simulink model "Correlation"  (R2012b)
settings: Solver=ode45  StartTime=0.0  StopTime=1280e-9  RelTol=1e-3
undefined symbols (not defined in the file or in its folder): Radix
libraries: dspxfrm3 x6
settings Model: Creator=Ahmad  LastModifiedBy=Ahmad

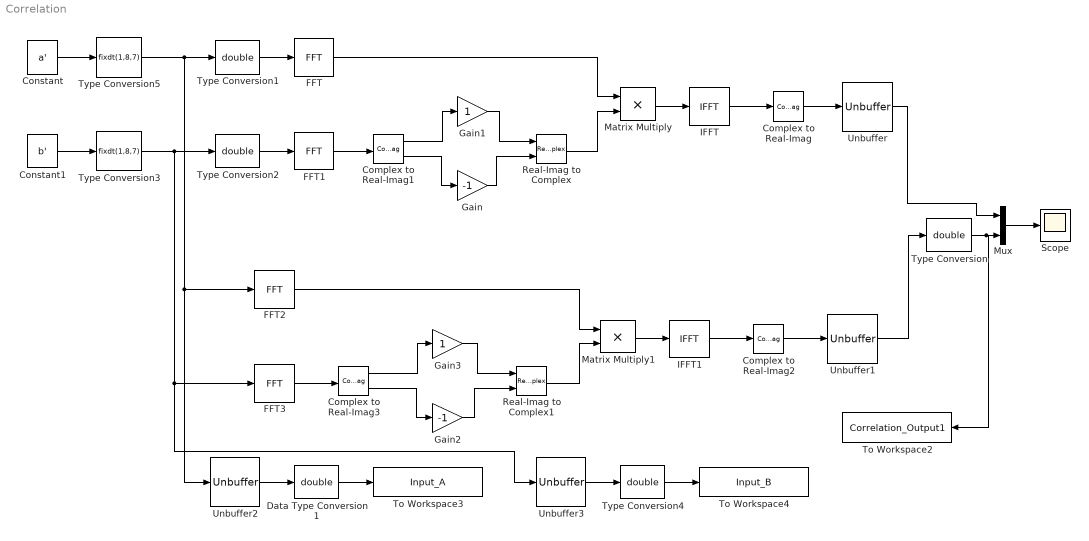
== system Correlation ==
  Complex to Real-Imag : ComplexToRealImag  Output=Real
  Complex to Real-Imag1 : ComplexToRealImag
  Complex to Real-Imag2 : ComplexToRealImag  Output=Real
  Complex to Real-Imag3 : ComplexToRealImag
  Constant : Constant  Value=a'  VectorParams1D=off  OutDataTypeStr=double  SampleTime=1/100e6  FramePeriod=128/100e6
      settings: SamplingMode=Frame based
  Constant1 : Constant  Value=b'  VectorParams1D=off  OutDataTypeStr=double  SampleTime=1/100e6  FramePeriod=128/100e6
      settings: SamplingMode=Frame based
  Data Type Conversion1 : DataTypeConversion  OutDataTypeStr=double
  FFT : dspxfrm3/FFT  CompMethod=Table lookup  TableOpt=NEW  TableOptActive=Speed  BitRevOrder=off  InheritFFTLength=off  FFTLength=128  RowConvenienceOn=on  FFTImplementation=Radix-2  SkipNorm=off  firstCoeffDataTypeStr=Inherit: Same word length as input  firstCoeffLastDataTypeStr=Inherit: Same word length as input  outputMin=[]  outputMax=[]  roundingMode=Floor  overflowMode=off
  FFT1 : dspxfrm3/FFT  CompMethod=Table lookup  TableOpt=NEW  TableOptActive=Speed  BitRevOrder=off  InheritFFTLength=off  FFTLength=128  RowConvenienceOn=on  FFTImplementation=Radix-2  SkipNorm=off  firstCoeffDataTypeStr=Inherit: Same word length as input  firstCoeffLastDataTypeStr=Inherit: Same word length as input  outputMin=[]  outputMax=[]  roundingMode=Floor  overflowMode=off
  FFT2 : dspxfrm3/FFT  CompMethod=Table lookup  TableOpt=NEW  TableOptActive=Speed  BitRevOrder=off  InheritFFTLength=off  FFTLength=128  RowConvenienceOn=on  FFTImplementation=Radix-2  SkipNorm=off  firstCoeffMode=Specify word length  firstCoeffWordLength=8  firstCoeffFracLength=15  firstCoeffDataTypeStr=fixdt(1,8)  firstCoeffLastDataTypeStr=fixdt(1,8)  outputMode=Binary point scaling  outputWordLength=16  outputFracLength=7  outputDataTypeStr=fixdt(1,16,7)  outputLastDataTypeStr=fixdt(1,16,7)  outputMin=[]  outputMax=[]  accumMode=Binary point scaling  accumWordLength=16  accumFracLength=7  accumDataTypeStr=fixdt(1,16,7)  accumLastDataTypeStr=fixdt(1,16,7)  prodOutputMode=Binary point scaling  prodOutputWordLength=11  prodOutputFracLength=7  prodOutputDataTypeStr=fixdt(1,11,7)  prodOutputLastDataTypeStr=fixdt(1,11,7)  roundingMode=Floor  overflowMode=off
  FFT3 : dspxfrm3/FFT  CompMethod=Table lookup  TableOpt=NEW  TableOptActive=Speed  BitRevOrder=off  InheritFFTLength=off  FFTLength=128  RowConvenienceOn=on  FFTImplementation=Radix-2  SkipNorm=off  firstCoeffMode=Specify word length  firstCoeffWordLength=8  firstCoeffFracLength=15  firstCoeffDataTypeStr=fixdt(1,8)  firstCoeffLastDataTypeStr=fixdt(1,8)  outputMode=Binary point scaling  outputWordLength=16  outputFracLength=7  outputDataTypeStr=fixdt(1,16,7)  outputLastDataTypeStr=fixdt(1,16,7)  outputMin=[]  outputMax=[]  accumMode=Binary point scaling  accumWordLength=16  accumFracLength=7  accumDataTypeStr=fixdt(1,16,7)  accumLastDataTypeStr=fixdt(1,16,7)  prodOutputMode=Binary point scaling  prodOutputWordLength=11  prodOutputFracLength=7  prodOutputDataTypeStr=fixdt(1,11,7)  prodOutputLastDataTypeStr=fixdt(1,11,7)  roundingMode=Floor  overflowMode=off
  Gain : Gain  Gain=-1
  Gain1 : Gain
  Gain2 : Gain  Gain=-1  OutDataTypeStr=fixdt(1,16,7)
  Gain3 : Gain  OutDataTypeStr=fixdt(1,16,7)
  IFFT : dspxfrm3/IFFT  CompMethod=Table lookup  TableOpt=NEW  TableOptActive=Speed  BitRevOrder=off  cs_in=off  SkipNorm=off  InheritFFTLength=off  FFTLength=128  mode=Complex  outSamplingMode=Frame based  RowConvenienceOn=on  FFTImplementation=Radix-2  firstCoeffDataTypeStr=Inherit: Same word length as input  firstCoeffLastDataTypeStr=Inherit: Same word length as input  outputMin=[]  outputMax=[]  roundingMode=Floor  overflowMode=off
  IFFT1 : dspxfrm3/IFFT  CompMethod=Table lookup  TableOpt=NEW  TableOptActive=Speed  BitRevOrder=off  cs_in=off  SkipNorm=off  InheritFFTLength=off  FFTLength=128  mode=Complex  outSamplingMode=Frame based  RowConvenienceOn=on  FFTImplementation=Radix-2  firstCoeffMode=Specify word length  firstCoeffWordLength=16  firstCoeffFracLength=15  firstCoeffDataTypeStr=fixdt(1,16)  firstCoeffLastDataTypeStr=fixdt(1,16)  outputMode=Binary point scaling  outputWordLength=33  outputFracLength=7  outputDataTypeStr=fixdt(1,33,7)  outputLastDataTypeStr=fixdt(1,33,7)  outputMin=[]  outputMax=[]  accumMode=Binary point scaling  accumWordLength=33  accumFracLength=7  accumDataTypeStr=fixdt(1,33,7)  accumLastDataTypeStr=fixdt(1,33,7)  prodOutputMode=Binary point scaling  prodOutputWordLength=25  prodOutputFracLength=7  prodOutputDataTypeStr=fixdt(1,25,7)  prodOutputLastDataTypeStr=fixdt(1,25,7)  roundingMode=Floor  overflowMode=off
  Matrix Multiply : Product
  Matrix Multiply1 : Product  OutDataTypeStr=fixdt(1,25,7)
  Mux : Mux  Inputs=2
  Real-Imag to Complex : RealImagToComplex
  Real-Imag to Complex1 : RealImagToComplex
  Scope : Scope
      settings: YMin=0.1  YMax=0.85
  To Workspace2 : ToWorkspace  VariableName=Correlation_Output1  SampleTime=-1  SaveFormat=Timeseries
  To Workspace3 : ToWorkspace  VariableName=Input_A  SampleTime=-1  SaveFormat=Timeseries
  To Workspace4 : ToWorkspace  VariableName=Input_B  SampleTime=-1  SaveFormat=Timeseries
  Type Conversion{,1..2,4} (4 alike) : DataTypeConversion  OutDataTypeStr=double
  Type Conversion3 : DataTypeConversion  OutDataTypeStr=fixdt(1,8,7)
  Type Conversion5 : DataTypeConversion  OutDataTypeStr=fixdt(1,8,7)
  Unbuffer{,1..3} (4 alike) : Unbuffer
  wires:
  Complex to Real-Imag/1 -> Unbuffer/1
  IFFT/1 -> Complex to Real-Imag/1
  FFT1/1 -> Complex to Real-Imag1/1
  Complex to Real-Imag1/1 -> Gain1/1
  Complex to Real-Imag1/2 -> Gain/1
  Gain1/1 -> Real-Imag to Complex/1
  Gain/1 -> Real-Imag to Complex/2
  FFT/1 -> Matrix Multiply/1
  Real-Imag to Complex/1 -> Matrix Multiply/2
  Matrix Multiply/1 -> IFFT/1
  Constant/1 -> Type Conversion5/1
  Constant1/1 -> Type Conversion3/1
  Unbuffer/1 -> Mux/1
  Complex to Real-Imag2/1 -> Unbuffer1/1
  IFFT1/1 -> Complex to Real-Imag2/1
  FFT3/1 -> Complex to Real-Imag3/1
  Complex to Real-Imag3/1 -> Gain3/1
  Complex to Real-Imag3/2 -> Gain2/1
  Gain3/1 -> Real-Imag to Complex1/1
  Gain2/1 -> Real-Imag to Complex1/2
  FFT2/1 -> Matrix Multiply1/1
  Matrix Multiply1/1 -> IFFT1/1
  Unbuffer1/1 -> Type Conversion/1
  Mux/1 -> Scope/1
  Type Conversion/1 -> To Workspace2/1, Mux/2
  Type Conversion1/1 -> FFT/1
  Type Conversion2/1 -> FFT1/1
  Data Type Conversion1/1 -> To Workspace3/1
  Type Conversion5/1 -> Type Conversion1/1, FFT2/1, Unbuffer2/1
  Type Conversion3/1 -> FFT3/1, Unbuffer3/1, Type Conversion2/1
  Unbuffer2/1 -> Data Type Conversion1/1
  Type Conversion4/1 -> To Workspace4/1
  Unbuffer3/1 -> Type Conversion4/1
  Real-Imag to Complex1/1 -> Matrix Multiply1/2
